simulink model "DCDC_SEPIC_TopLevelModel_HW"  (R2024b)
settings: configuration reference "ConfigSet_HW_ASW" (kept outside this file)
PostLoadFcn:
  | obj=getActiveConfigSet(mdlNames.topLevel);
  | if ~strcmp(obj.Name, 'Ref_ConfigSet_HW_ASW')
  | VoltCL_LEDCL_TIHardware;
  | end
settings Model: DataDictionary=LocalDataD_TopLevelModelData.sldd  SimulationMode=external  Creator=vlenzi  LastModifiedBy=vlenzi
settings ConfigSetRef: SourceName=ConfigSet_HW_ASW

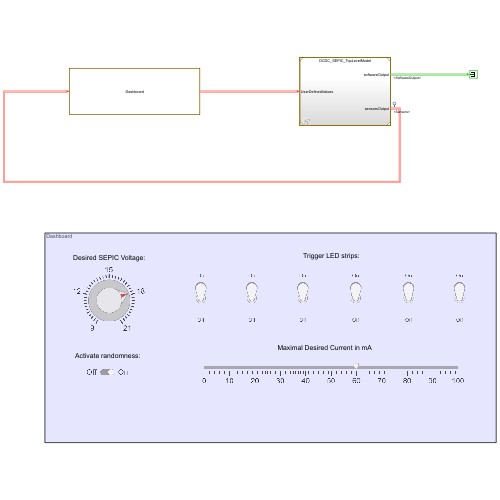
[thumbnail: Simulink's stored preview of the top-level diagram]
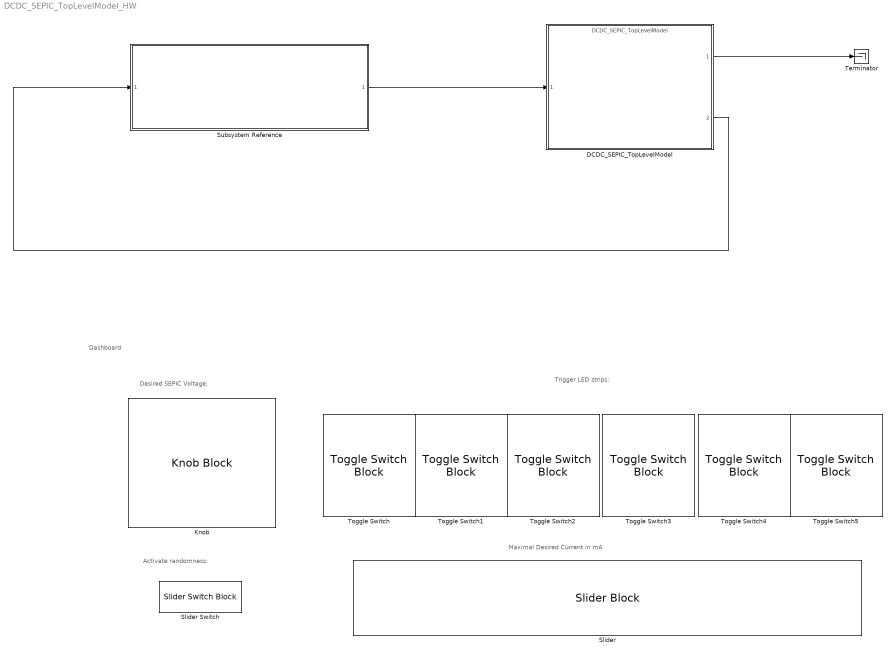
== system DCDC_SEPIC_TopLevelModel_HW ==
  note: Trigger LED strips:
  note: Maximal Desired Current in mA
  note: Dashboard
  note: Activate randomness:
  note: Desired SEPIC Voltage:
  DCDC_SEPIC_TopLevelModel : ModelReference  ModelNameDialog=DCDC_SEPIC_TopLevelModel  SimulationMode=Normal  ModelReferenceVersion=10.17
  Knob : KnobBlock  LabelPosition=Hide  ScaleMin=9  ScaleMax=21  TickInterval=3
  Slider : SliderBlock  LabelPosition=Hide  TickInterval=10
  Slider Switch : SliderSwitchBlock  LabelPosition=Hide
      settings: Values={{'Off', 'On'}, [0 1]}
  Subsystem Reference : Subsystem  ReferencedSubsystem=User_Interface_Dashboard
  Terminator : Terminator
  Toggle Switch{,1..5} (6 alike) : ToggleSwitchBlock  LabelPosition=Hide
      settings: Values={{'Off', 'On'}, [0 1]}
  wires:
  Subsystem Reference/1 -> DCDC_SEPIC_TopLevelModel/1
  DCDC_SEPIC_TopLevelModel/2 -> Subsystem Reference/1
  DCDC_SEPIC_TopLevelModel/1 -> Terminator/1
